simulink model "project_3_ic"  (R2013b)
settings: Solver=ode45  StartTime=0.0  StopTime=50  RelTol=1e-3
settings Model: Creator=neel  LastModifiedBy=ANCHE BHANU THEJA
settings DataIOCC: SignalLoggingSaveFormat=ModelDataLogs
settings OptimizationCC: ExpressionDepthLimit=2147483647
settings DebuggingCC: MultiTaskDSMMsg=warning  MultiTaskCondExecSysMsg=none  StateNameClashWarn=warning
settings RTWCC: IncludeERTFirstTime=on
settings GRTTargetCC: CodeReplacementLibrary=None  CPPClassGenCompliant=on

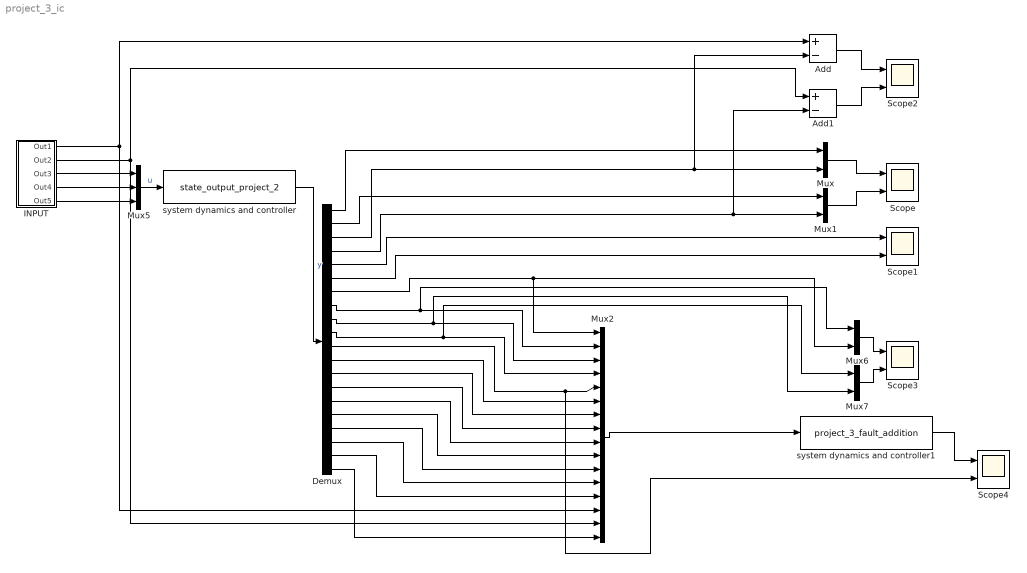
== system project_3_ic ==
  Add : Sum  Inputs=+-
  Add1 : Sum  Inputs=+-
  Demux : Demux  Outputs=20
  INPUT : Subsystem
  Mux{,1,6..7} (4 alike) : Mux  Inputs=2
  Mux2 : Mux  Inputs=16
  Mux5 : Mux  Inputs=3
  Scope{,1..4} (5 alike) : Scope  NumInputPorts=2
      Scope settings: YMin=-5~-5  YMax=5~5
      Scope1 settings: YMin=-5~-5  YMax=5~5
      Scope2 settings: YMin=-5~-5  YMax=5~5  SaveName=ScopeData2
      Scope3 settings: YMin=2.09715e+06~4.1943e+06  YMax=3.5e+22~7e+22  SaveName=ScopeData3
      Scope4 settings: YMin=-5~-5  YMax=5~5  SaveName=ScopeData4
  system dynamics and controller : S-Function  FunctionName=state_output_project_2  EnableBusSupport=off
  system dynamics and controller1 : S-Function  FunctionName=project_3_fault_addition  EnableBusSupport=off
  wires:
  Mux1/1 -> Scope/2
  Mux5/1 -> system dynamics and controller/1  "u"
  Add/1 -> Scope2/1
  Add1/1 -> Scope2/2
  Mux/1 -> Scope/1
  Mux6/1 -> Scope3/1
  Mux7/1 -> Scope3/2
  INPUT/1(Out1) -> Mux2/14, Add/1
  INPUT/2(Out2) -> Mux2/15, Add1/1
  INPUT/3(Out3) -> Mux5/1
  INPUT/4(Out4) -> Mux5/2
  INPUT/5(Out5) -> Mux5/3
  system dynamics and controller1/1 -> Scope4/1
  Demux/10 -> Mux2/4, Mux7/1
  Demux/4 -> Mux1/2, Add1/2
  Demux/2 -> Mux1/1
  Demux/7 -> Mux2/1, Mux6/2
  Demux/8 -> Mux2/2, Mux6/1
  Demux/9 -> Mux2/3, Mux7/2
  system dynamics and controller/1 -> Demux/1  "y"
  Demux/1 -> Mux/1
  Demux/3 -> Mux/2, Add/2
  Demux/5 -> Scope1/1
  Demux/6 -> Scope1/2
  Demux/11 -> Scope4/2, Mux2/5
  Demux/12 -> Mux2/6
  Demux/13 -> Mux2/7
  Demux/14 -> Mux2/8
  Demux/15 -> Mux2/9
  Demux/16 -> Mux2/10
  Demux/17 -> Mux2/11
  Demux/18 -> Mux2/12
  Demux/19 -> Mux2/13
  Mux2/1 -> system dynamics and controller1/1
  Demux/20 -> Mux2/16

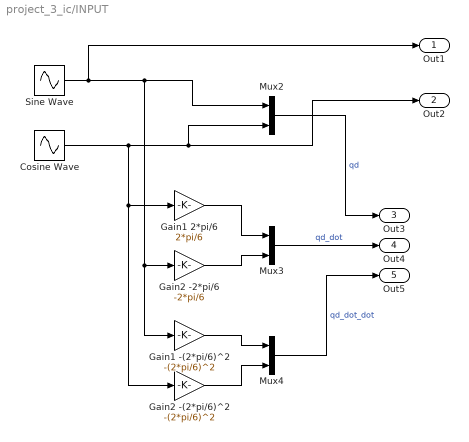
== system project_3_ic/INPUT ==
  Cosine Wave : Sin  Amplitude=0.2  Frequency=2*pi/6  Phase=pi/2  SampleTime=0
  Gain1 -(2*pi/6)^2 : Gain  Gain=-(2*pi/6)^2
  Gain1 2*pi/6 : Gain  Gain=2*pi/6
  Gain2 -(2*pi/6)^2 : Gain  Gain=-(2*pi/6)^2
  Gain2 -2*pi/6 : Gain  Gain=-2*pi/6
  Mux2 : Mux  Inputs=2
  Mux3 : Mux  Inputs=2
  Mux4 : Mux  Inputs=2
  Sine Wave : Sin  Amplitude=0.2  Frequency=2*pi/6  SampleTime=0
  Out1 : Outport
  Out2 : Outport  Port=2
  Out3 : Outport  Port=3
  Out4 : Outport  Port=4
  Out5 : Outport  Port=5
  wires:
  Mux4/1 -> Out5/1  "qd_dot_dot"
  Cosine Wave/1 -> Out2/1, Mux2/2, Gain2 -(2*pi/6)^2/1, Gain1 2*pi/6/1
  Gain1 -(2*pi/6)^2/1 -> Mux4/1
  Gain2 -(2*pi/6)^2/1 -> Mux4/2
  Gain2 -2*pi/6/1 -> Mux3/2
  Gain1 2*pi/6/1 -> Mux3/1
  Mux3/1 -> Out4/1  "qd_dot"
  Mux2/1 -> Out3/1  "qd"
  Sine Wave/1 -> Out1/1, Gain1 -(2*pi/6)^2/1, Gain2 -2*pi/6/1, Mux2/1
